simulink model "HealthRequestDecoder"  (R2023a)
settings: Solver=VariableStepAuto  StartTime=0.0  StopTime=10.0  RelTol=1e-3
undefined symbols (not defined in the file): I, OReq
settings Model: Creator=aan18022  LastModifiedBy=aan18022

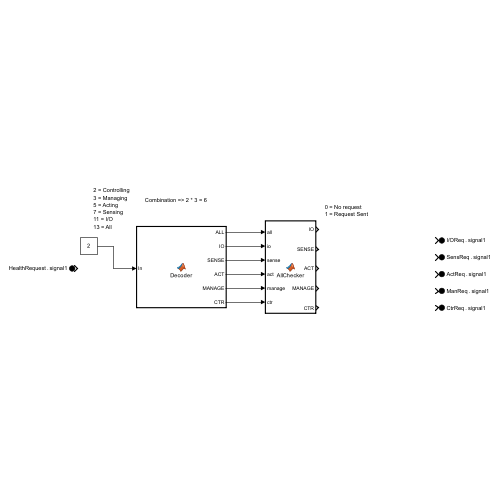
[thumbnail: Simulink's stored preview of the top-level diagram]
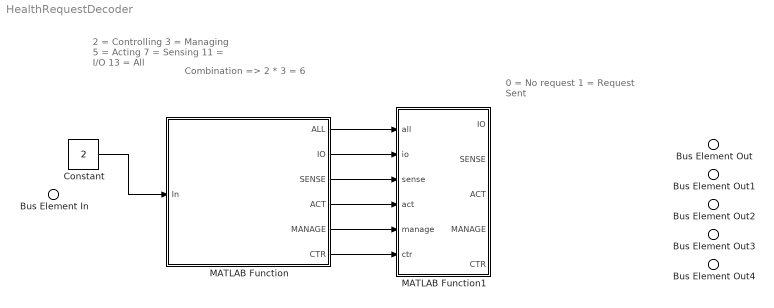
== system HealthRequestDecoder ==
  note: 0 = No request
      | 1 = Request Sent
  note: Combination => 2 * 3 = 6
  note: 2 = Controlling
      | 3 = Managing
      | 5 = Acting
      | 7 = Sensing
      | 11 = I/O
      | 13 = All
  Bus Element In : Inport  PortName=HealthRequest  Element=signal1
  Constant : Constant  Value=2
  MATLAB Function : MATLAB Function  TreatAsAtomicUnit=on
  MATLAB Function1 : MATLAB Function  TreatAsAtomicUnit=on
  Bus Element Out : Outport  PortName=I/OReq  Element=signal1
  Bus Element Out1 : Outport  Port=2  PortName=SensReq  Element=signal1
  Bus Element Out2 : Outport  Port=3  PortName=ActReq  Element=signal1
  Bus Element Out3 : Outport  Port=4  PortName=ManReq  Element=signal1
  Bus Element Out4 : Outport  Port=5  PortName=CtrReq  Element=signal1
  wires:
  MATLAB Function/2(IO) -> MATLAB Function1/2(io)
  MATLAB Function/4(ACT) -> MATLAB Function1/4(act)
  MATLAB Function/5(MANAGE) -> MATLAB Function1/5(manage)
  MATLAB Function/1(ALL) -> MATLAB Function1/1(all)
  MATLAB Function/6(CTR) -> MATLAB Function1/6(ctr)
  MATLAB Function/3(SENSE) -> MATLAB Function1/3(sense)
  Constant/1 -> MATLAB Function/1(In)

== matlab function HealthRequestDecoder/MATLAB Function1 ==
  data: all input; IO output; io input; sense input; act input; manage input; ctr input; SENSE output; ACT output; MANAGE output; CTR output
function [IO,SENSE,ACT,MANAGE,CTR]= AllChecker(all,io,sense,act,manage,ctr)

if (all == 1)
    IO = 1;
    SENSE = 1;
    ACT = 1;
    MANAGE = 1;
    CTR = 1;
else
    IO = io;
    SENSE = sense;
    ACT = act;
    MANAGE = manage;
    CTR = ctr;
end

== matlab function HealthRequestDecoder/MATLAB Function ==
  data: In input; ALL output; IO output; SENSE output; ACT output; MANAGE output; CTR output
function [ALL,IO,SENSE,ACT,MANAGE,CTR]= Decoder(In)

al = mod(In,13);%All
io  = mod(In,11);
s  = mod(In,7);
ac = mod(In,5);
m  = mod(In,3);
c  = mod(In,2);

if (al == 0)
    ALL = 1;
else
    ALL = 0;
end

if (io == 0)
    IO = 1;
else
    IO = 0;
end

if (s == 0)
    SENSE = 1;
else
    SENSE = 0;
end

if (ac == 0)
    ACT = 1;
else
    ACT = 0;    
end

if (m == 0)
    MANAGE = 1;
else
    MANAGE = 0;
end

if (c == 0)
    CTR = 1;
else
    CTR = 0;
end
